simulink model "vipwarningsigns"  (R2017b)
settings: Solver=FixedStepDiscrete  StartTime=0  StopTime=inf  RelTol=1e-3  EnableMultiTasking=on
InitFcn:
  | % Maximum number of signs in a single frame
  | maxNumSigns=9;
  | % The .mat file reference below was generated using vipwarningsigns_templates.m
  | load vipwarningsigns_templates.mat;
model workspace (MATLAB code in the model file):
  | MaxBlkWidth=80;
undefined symbols (not defined in the file or in its folder): gray, Rec, SDTV, strel, template_detection, template_detection_display, template_ids, template_names, template_recognition, template_recognition_display
libraries: simulink x4, visiontextngfix x3, visionstatistics x1, visionmorphops x1, vipmisc x1, visionconversions x1, dspvision x1
CloseFcn:
  | clear maxNumSigns;
  | clear template_detection;
  | clear template_detection_display;
  | clear template_ids;
  | clear template_names;
  | clear template_recognition;
  | clear template_recognition_display;
settings Model: FPTRunName=Active  ExtModeAutoUpdateStatusClock=off  Creator=The MathWorks, Inc.  LastModifiedBy=The MathWorks, Inc.
settings DataIOCC: LimitDataPoints=on  SaveFormat=Array  SaveOutput=off  SignalLogging=off  SaveTime=off
settings OptimizationCC: ExpressionDepthLimit=2147483647  InitFltsAndDblsToZero=on  EfficientMapNaN2IntZero=off  LifeSpan=inf
settings DebuggingCC: UnderspecifiedInitializationDetection=Classic  MergeDetectMultiDrivingBlocksExec=none  SignalResolutionControl=TryResolveAllWithWarning  SolverPrmCheckMsg=warning  MultiTaskDSMMsg=warning  MultiTaskCondExecSysMsg=none  SigSpecEnsureSampleTimeMsg=none  ParameterPrecisionLossMsg=none  FcnCallInpInsideContextMsg=warning  AllowSymbolicDim=off  StateNameClashWarn=warning  SFUnexpectedBacktrackingDiag=warning  SFNoUnconditionalDefaultTransitionDiag=warning  SFExecutionAtInitializationDiag=none
settings HardwareCC: ProdBitPerPointer=32  ProdBitPerSizeT=32  ProdBitPerPtrDiffT=32  ProdLargestAtomicFloat=None  ProdIntDivRoundTo=Undefined  ProdEndianess=Unspecified  ProdWordSize=32  ProdHWDeviceType=32-bit Generic
settings ModelReferenceCC: PropagateSignalLabelsOutOfModel=off
settings SFSimCC: SimParseCustomCode=off
settings CodeAppCC: StateflowObjectComments=on
settings GRTTargetCC: TargetLangStandard=C89/C90 (ANSI)  GeneratePreprocessorConditionals=Disable all  CombineOutputUpdateFcns=off  GRTInterface=on
settings ConfigComp: CovMetricSettings=dw  CovHtmlReporting=on  CovSaveCumulativeToWorkspaceVar=on  CovSaveSingleToWorkspaceVar=on  CovExternalEMLEnable=off

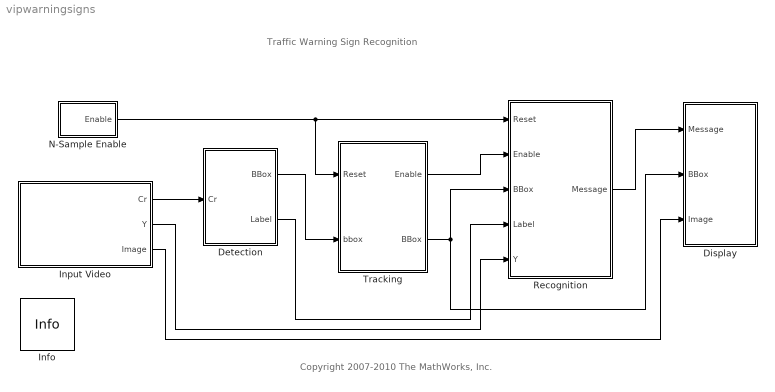
== system vipwarningsigns ==
  note: Traffic Warning Sign Recognition
  note: Copyright 2007-2010 The MathWorks, Inc.
  Detection : Subsystem
  Display : Subsystem
  Info : vipmisc/Info  SystemSampleTime=-1
      settings: SourceProductName=Computer Vision System Toolbox  SourceProductBaseCode=VP
  Input Video : Subsystem
      mask Display:
      | disp('vipwarnsigns.avi');
      | port_label('output',1,'Cr');
      | port_label('output',2,'Y');
      | port_label('output',3,'Image');
  N-Sample Enable : Subsystem  mask{sample=1}
      mask prompts: sample "Trigger Count, N"
  Recognition : Subsystem
  Tracking : Subsystem
  wires:
  Detection/1(BBox) -> Tracking/2(bbox)
  Input Video/1(Cr) -> Detection/1(Cr)
  N-Sample Enable/1(Enable) -> Tracking/1(Reset), Recognition/1(Reset)
  Tracking/1(Enable) -> Recognition/2(Enable)
  Tracking/2(BBox) -> Recognition/3(BBox), Display/2(BBox)
  Detection/2(Label) -> Recognition/4(Label)
  Input Video/2(Y) -> Recognition/5(Y)
  Recognition/1(Message) -> Display/1(Message)
  Input Video/3(Image) -> Display/3(Image)

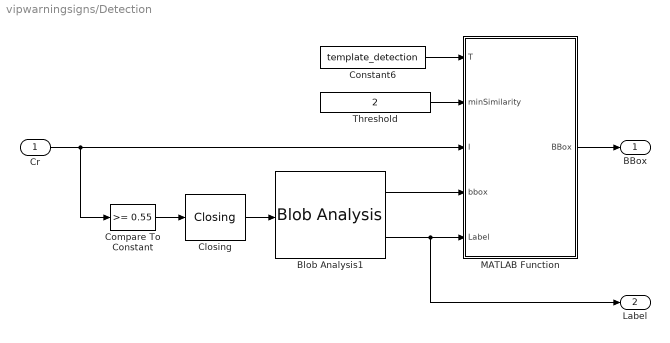
== system vipwarningsigns/Detection ==
  Cr : Inport
  Blob Analysis1 : visionstatistics/Blob Analysis  Tag=vipblks_row_conv  area=off  centroid=off  bBox=on  majorAxis=off  minorAxis=off  angle=off  eccentricity=off  equivDiameterSq=off  extent=off  perimeter=off  maxBlobs=maxNumSigns  warnIfNumBlobsExceeded=on  isCount=off  useMinArea=off  minArea=0  useMaxArea=off  maxArea=intmax('uint32')  excludeBorderBlob=off  outDT=double  isOutVarDim=on  isFill=on  fillValues=-1  conn=8  isLabel=on  outputMode=Binary point scaling  outputWordLength=32  outputFracLength=16  firstCoeffMode=Binary point scaling  firstCoeffWordLength=16  firstCoeffFracLength=14  secondCoeffMode=Binary point scaling  secondCoeffWordLength=32  secondCoeffFracLength=16  accumMode=Binary point scaling  accumWordLength=32  accumFracLength=0  prodOutputMode=Binary point scaling  prodOutputWordLength=32  prodOutputFracLength=16  roundingMode=Floor  overflowMode=off
      settings: SourceProductName=Computer Vision System Toolbox
  Closing : visionmorphops/Closing  nhoodsrc=Specify via dialog  strel=strel('rectangle', [15 15])
      settings: SourceProductName=Computer Vision System Toolbox  SourceProductBaseCode=VP
  Compare To Constant : simulink/Logic and Bit Operations/Compare To Constant  relop=>=  const=0.55  OutDataTypeStr=boolean  ZeroCross=off
  Constant6 : Constant  Value=template_detection  OutDataTypeStr=single
  MATLAB Function : MATLAB Function  TreatAsAtomicUnit=on
  Threshold : Constant  Value=2  OutDataTypeStr=single
  BBox : Outport
  Label : Outport  Port=2
  wires:
  Cr/1 -> MATLAB Function/3(I), Compare To Constant/1
  Closing/1 -> Blob Analysis1/1
  MATLAB Function/1(BBox) -> BBox/1
  Constant6/1 -> MATLAB Function/1(T)
  Blob Analysis1/2 -> MATLAB Function/5(Label), Label/1
  Compare To Constant/1 -> Closing/1
  Threshold/1 -> MATLAB Function/2(minSimilarity)
  Blob Analysis1/1 -> MATLAB Function/4(bbox)

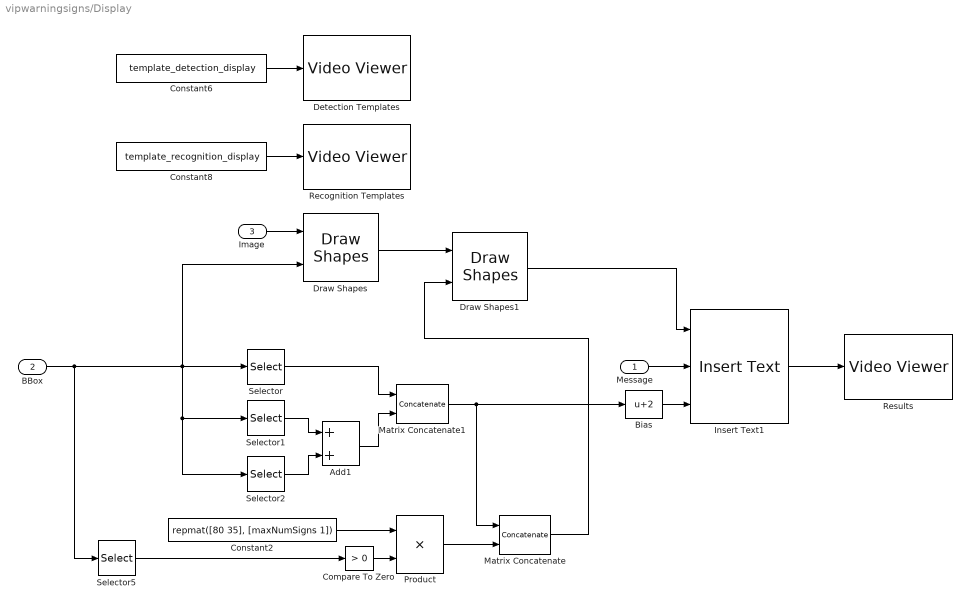
== system vipwarningsigns/Display ==
  Message : Inport
  BBox : Inport  Port=2
  Image : Inport  Port=3
  Add1 : Sum
  Bias : Bias  Bias=2
  Compare To Zero : simulink/Logic and Bit Operations/Compare To Zero  relop=>  OutDataTypeStr=uint8  ZeroCross=off
  Constant2 : Constant  Value=repmat([80 35], [maxNumSigns 1])  VectorParams1D=off  OutDataTypeStr=single
  Constant6 : Constant  Value=template_detection_display  OutDataTypeStr=single
  Constant8 : Constant  Value=template_recognition_display  OutDataTypeStr=single
  Detection Templates : VideoViewer  colormapValue=gray(256)  FigPos=[200 158 371 65]
  Draw Shapes : visiontextngfix/Draw Shapes  shape=Rectangles  fill=off  lineWidth=1  fillClrSource=Specify via dialog  display=User-specified value  intensity=200  color=[1 1 0]  opacity=0.6  viewport=Entire image  antialiasing=off  inType=Obsolete  imagePorts=One multidimensional signal  prodOutputMode=Binary point scaling  prodOutputWordLength=32  prodOutputFracLength=14  memoryMode=Specify word length  memoryWordLength=16  memoryFracLength=15  roundingMode=Floor  overflowMode=off
      settings: SourceProductName=Computer Vision System Toolbox
  Draw Shapes1 : visiontextngfix/Draw Shapes  shape=Rectangles  fill=on  lineWidth=1  fillClrSource=Specify via dialog  display=User-specified value  intensity=200  color=single([0 0 0])  opacity=single(1)  viewport=Entire image  antialiasing=off  inType=Obsolete  imagePorts=One multidimensional signal  prodOutputMode=Binary point scaling  prodOutputWordLength=32  prodOutputFracLength=14  memoryMode=Specify word length  memoryWordLength=16  memoryFracLength=14  roundingMode=Floor  overflowMode=off
      settings: SourceProductName=Computer Vision System Toolbox
  Insert Text1 : visiontextngfix/Insert Text  inputType=Obsolete  theText='%s'  getTextLocFrom=Input port  textLoc=[0 0]  getTextColorFrom=Specify via dialog  textColor=[1 0 0]'  getTextIntensityFrom=Specify via dialog  textIntensity=0  getTextOpacityFrom=Specify via dialog  textOpacity=1.0  dummyVar2=0  dummyVar3=0  dummyVar4=0  imagePorts=One multidimensional signal  isInputTransposed=off  fontFace=LucidaSansRegular  dummyVar1=0  blockFontSize=12  antiAliased=on
      settings: SourceProductName=Computer Vision System Toolbox  SourceProductBaseCode=VP
  Matrix Concatenate : Concatenate  Mode=Multidimensional array  ConcatenateDimension=2
  Matrix Concatenate1 : Concatenate  Mode=Multidimensional array  ConcatenateDimension=2
  Product : Product  RndMeth=Zero
  Recognition Templates : VideoViewer  colormapValue=gray(256)  FigPos=[200 325 371 88]
  Results : VideoViewer  colormapValue=gray(256)  FigPos=[585 365 410 238]
  Selector : Selector  NumberOfDimensions=2  InputPortWidth=4  IndexOptions=Select all,Index vector (dialog)  Indices=1,1  OutputSizes=1,1
  Selector1 : Selector  NumberOfDimensions=2  InputPortWidth=4  IndexOptions=Select all,Index vector (dialog)  Indices=3,2  OutputSizes=1,1
  Selector2 : Selector  NumberOfDimensions=2  InputPortWidth=4  IndexOptions=Select all,Index vector (dialog)  Indices=2,4  OutputSizes=1,1
  Selector5 : Selector  NumberOfDimensions=2  InputPortWidth=4  IndexOptions=Select all,Index vector (dialog)  Indices=[3 4],[3 4]  OutputSizes=1,1
  wires:
  Message/1 -> Insert Text1/2
  Image/1 -> Draw Shapes/1
  Insert Text1/1 -> Results/1
  Bias/1 -> Insert Text1/3
  Constant6/1 -> Detection Templates/1
  Constant8/1 -> Recognition Templates/1
  Selector/1 -> Matrix Concatenate1/1
  Selector1/1 -> Add1/1
  Draw Shapes/1 -> Draw Shapes1/1
  Draw Shapes1/1 -> Insert Text1/1
  Matrix Concatenate1/1 -> Bias/1, Matrix Concatenate/1
  Product/1 -> Matrix Concatenate/2
  Matrix Concatenate/1 -> Draw Shapes1/2
  Compare To Zero/1 -> Product/2
  Constant2/1 -> Product/1
  Selector5/1 -> Compare To Zero/1
  BBox/1 -> Selector5/1, Selector1/1, Selector2/1, Selector/1, Draw Shapes/2
  Selector2/1 -> Add1/2
  Add1/1 -> Matrix Concatenate1/2

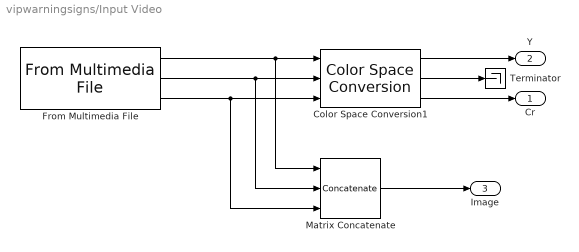
== system vipwarningsigns/Input Video ==
  Color Space Conversion1 : visionconversions/Color Space  Conversion  conversion=Obsolete  conversionActive=R'G'B' to Y'CbCr  wp_str=D65  rec=Rec. 601 (SDTV)  sys=1125/60/2:1  imagePorts=Separate color signals
      settings: SourceProductName=Computer Vision System Toolbox
  From Multimedia File : dspvision/From Multimedia File  inputFilename=vipwarnsigns.avi  loop=on  numPlays=inf  outputStreams=Video and audio  videoDataType=single  audioDataType=int16  inheritSampleTime=on  userDefinedSampleTime=1/30  noAudioOutput=off  isIntensityVideo=off  fourcc=RGB  colorVideoFormat=Separate color signals  outputEOF=off  dataOrg=Column-major  audioFrameSize=1024  computeAudioFrameSize=off  outSamplingMode=Frame based
      settings: SourceProductBaseCode=VP
  Matrix Concatenate : Concatenate  NumInputs=3  Mode=Multidimensional array  ConcatenateDimension=3
  Terminator : Terminator
  Cr : Outport
  Y : Outport  Port=2
  Image : Outport  Port=3
  wires:
  From Multimedia File/1 -> Color Space Conversion1/1, Matrix Concatenate/1
  From Multimedia File/2 -> Color Space Conversion1/2, Matrix Concatenate/2
  From Multimedia File/3 -> Color Space Conversion1/3, Matrix Concatenate/3
  Color Space Conversion1/1 -> Y/1
  Color Space Conversion1/2 -> Terminator/1
  Color Space Conversion1/3 -> Cr/1
  Matrix Concatenate/1 -> Image/1

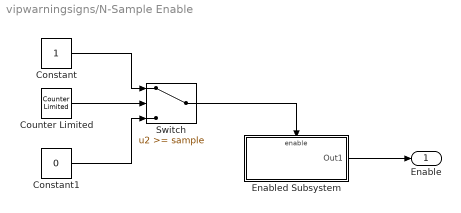
== system vipwarningsigns/N-Sample Enable ==
  Constant : Constant  OutDataTypeStr=boolean
  Constant1 : Constant  Value=0  OutDataTypeStr=boolean
  Counter Limited : simulink/Sources/Counter Limited  uplimit=sample  tsamp=-1
  Enabled Subsystem : Subsystem  TreatAsAtomicUnit=on
  Switch : Switch  Threshold=sample
  Enable : Outport
  wires:
  Counter Limited/1 -> Switch/2
  Constant1/1 -> Switch/3
  Constant/1 -> Switch/1
  Switch/1 -> Enabled Subsystem/Enable
  Enabled Subsystem/1(Out1) -> Enable/1

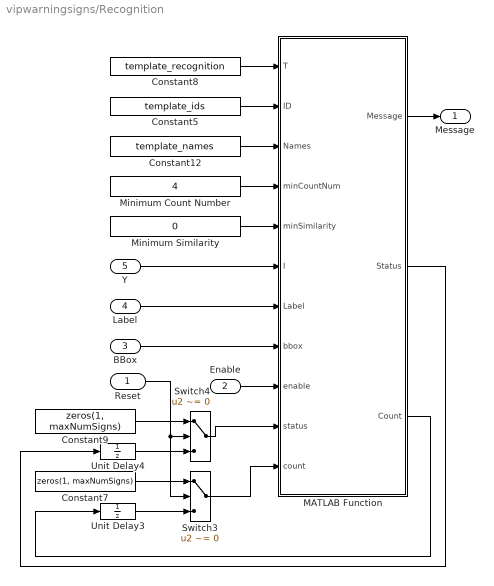
== system vipwarningsigns/Recognition ==
  Reset : Inport
  Enable : Inport  Port=2
  BBox : Inport  Port=3
  Label : Inport  Port=4
  Y : Inport  Port=5
  Constant12 : Constant  Value=template_names  OutDataTypeStr=single
  Constant5 : Constant  Value=template_ids  OutDataTypeStr=single
  Constant7 : Constant  Value=zeros(1, maxNumSigns)  OutDataTypeStr=single
  Constant8 : Constant  Value=template_recognition  OutDataTypeStr=single
  Constant9 : Constant  Value=zeros(1, maxNumSigns)  OutDataTypeStr=single
  MATLAB Function : MATLAB Function  TreatAsAtomicUnit=on
  Minimum Count Number : Constant  Value=4  OutDataTypeStr=single
  Minimum Similarity : Constant  Value=0  OutDataTypeStr=single
  Switch3 : Switch  Criteria=u2 ~= 0  OutDataTypeStr=Inherit: Inherit via back propagation  InputSameDT=on
  Switch4 : Switch  Criteria=u2 ~= 0  OutDataTypeStr=Inherit: Inherit via back propagation  InputSameDT=on
  Unit Delay3 : UnitDelay  SampleTime=-1
  Unit Delay4 : UnitDelay  SampleTime=-1
  Message : Outport
  wires:
  Constant8/1 -> MATLAB Function/1(T)
  Enable/1 -> MATLAB Function/9(enable)
  Y/1 -> MATLAB Function/6(I)
  MATLAB Function/1(Message) -> Message/1
  Reset/1 -> Switch3/2, Switch4/2
  BBox/1 -> MATLAB Function/8(bbox)
  Label/1 -> MATLAB Function/7(Label)
  Constant5/1 -> MATLAB Function/2(ID)
  Constant12/1 -> MATLAB Function/3(Names)
  MATLAB Function/2(Status) -> Unit Delay4/1
  Switch4/1 -> MATLAB Function/10(status)
  Unit Delay4/1 -> Switch4/3
  Constant9/1 -> Switch4/1
  MATLAB Function/3(Count) -> Unit Delay3/1
  Switch3/1 -> MATLAB Function/11(count)
  Unit Delay3/1 -> Switch3/3
  Constant7/1 -> Switch3/1
  Minimum Count Number/1 -> MATLAB Function/4(minCountNum)
  Minimum Similarity/1 -> MATLAB Function/5(minSimilarity)

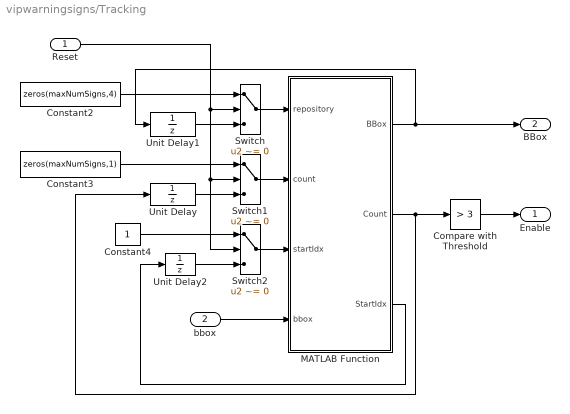
== system vipwarningsigns/Tracking ==
  Reset : Inport
  bbox : Inport  Port=2
  Compare with Threshold : simulink/Logic and Bit Operations/Compare To Constant  relop=>  const=3  OutDataTypeStr=boolean  ZeroCross=off
  Constant2 : Constant  Value=zeros(maxNumSigns,4)  OutDataTypeStr=single
  Constant3 : Constant  Value=zeros(maxNumSigns,1)  OutDataTypeStr=single
  Constant4 : Constant  OutDataTypeStr=single
  MATLAB Function : MATLAB Function  TreatAsAtomicUnit=on
  Switch : Switch  Criteria=u2 ~= 0  Threshold=1  OutDataTypeStr=Inherit: Inherit via back propagation  InputSameDT=on
  Switch1 : Switch  Criteria=u2 ~= 0  InputSameDT=on
  Switch2 : Switch  Criteria=u2 ~= 0  InputSameDT=on
  Unit Delay : UnitDelay  SampleTime=-1
  Unit Delay1 : UnitDelay  SampleTime=-1
  Unit Delay2 : UnitDelay  SampleTime=-1
  Enable : Outport
  BBox : Outport  Port=2
  wires:
  bbox/1 -> MATLAB Function/4(bbox)
  Compare with Threshold/1 -> Enable/1
  Reset/1 -> Switch2/2, Switch1/2, Switch/2
  Switch2/1 -> MATLAB Function/3(startIdx)
  MATLAB Function/3(StartIdx) -> Unit Delay2/1
  Unit Delay2/1 -> Switch2/3
  Constant4/1 -> Switch2/1
  Constant3/1 -> Switch1/1
  Unit Delay/1 -> Switch1/3
  MATLAB Function/2(Count) -> Compare with Threshold/1, Unit Delay/1
  MATLAB Function/1(BBox) -> BBox/1, Unit Delay1/1
  Unit Delay1/1 -> Switch/3
  Constant2/1 -> Switch/1
  Switch1/1 -> MATLAB Function/2(count)
  Switch/1 -> MATLAB Function/1(repository)

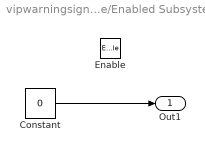
== system vipwarningsigns/N-Sample Enable/Enabled Subsystem ==
  Enable : EnablePort
  Constant : Constant  Value=0  OutDataTypeStr=boolean
  Out1 : Outport  InitialOutput=1
  wires:
  Constant/1 -> Out1/1

== matlab function vipwarningsigns/Tracking/MATLAB Function ==
  data: BBox output; repository input; count input; startIdx input; bbox input; Count output; StartIdx output; maxNumSigns parameter single size=1
function [BBox, Count, StartIdx] = Match(repository, count, startIdx, bbox, maxNumSigns)
% This function matches the targets found in the current video frame with
% those found in the previous frame. Targets in two video frames match
% when their bounding boxes overlap.
%
% Input:
%    repository: 
%       Bounding boxes of the targets found in the previous
%       frame. Each column has the format of [r, c, h, w] and corresponds 
%       to a target.
%    count: 
%       Number of video frames the target in the previous frame has 
%       been found.
%    startIdx: 
%       Index for the first new target in the current frame.
%    bbox: 
%       Bounding boxes of the targets found in the current frame.
%
% Output:
%    BBox: 
%       Bounding boxes of the targets found in the current frame. They
%       are ordered to have the same indices as their matching ones in the
%       previous frame.
%    Count: 
%       Number of video frames the target in the current frame has 
%       been found.
%    StartIdx: 
%       Index for the first new target in the next frame.

numBBox = single(size(bbox, 1));
BBox = single(zeros(maxNumSigns, 4));
Count = single(zeros(maxNumSigns,1));
impossible = single(10000); % A very large value
thr = single(2);
disMatrix = single(ones(maxNumSigns, numBBox)) * impossible;

% Calculate the distances between the repository and the current targets
for idx = single(1): maxNumSigns
    if repository(idx,3)>0 && repository(idx,4)>0
        for jdx = 1: numBBox
            if bbox(jdx,3)>0 && bbox(jdx,4)>0
                disMatrix(idx, jdx)...
                    = single(abs(2*(repository(idx,1)-bbox(jdx,1))...
                        +repository(idx,3)-bbox(jdx,3))...
                        / (repository(idx,3)+bbox(jdx,3))...
                        + abs(2*(repository(idx,2)-bbox(jdx,2))...
                        +repository(idx,4)-bbox(jdx,4))...
                        / (repository(idx,4)+bbox(jdx,4)));
            end
        end
    end
end

% Find the most similar pair of corners
for n = single(1): numBBox
    minVal = impossible;
    minIdx = single(0);
    minJdx = single(0);
    for idx = 1: single(maxNumSigns)
        for jdx = 1: numBBox
            if disMatrix(idx, jdx) < minVal
                minVal = disMatrix(idx, jdx);
                minIdx = idx;
                minJdx = jdx;
            end
        end
    end
    
    % Move the targets in the current frame so they have the same ordering
    % as their matching ones in the previous frame.
    if minVal < thr
        disMatrix(minIdx, :) = impossible;
        disMatrix(:, minJdx) = impossible;
        BBox(minIdx,:) = bbox(minJdx,:);
        Count(minIdx) = count(minIdx) + 1;
        bbox(minJdx,:) = single(zeros(4, 1));
    else
        break;
    end
end

% Copy the new targets
StartIdx = startIdx;
for jdx = single(1): numBBox
    if bbox(jdx,3)>0
        while BBox(StartIdx,3)
            if StartIdx<maxNumSigns
                StartIdx = StartIdx + single(1);
            else
                StartIdx = single(1);
            end
        end
        BBox(StartIdx, :) = bbox(jdx,:);
        Count(StartIdx) = single(1);
        if StartIdx<maxNumSigns
            StartIdx = StartIdx + single(1);
        else
            StartIdx = single(1);
        end
    end
end

== matlab function vipwarningsigns/Recognition/MATLAB Function ==
  data: Message output; Status output; T input; ID input; Names input; minCountNum input; minSimilarity input; I input; Label input; bbox input; enable input; status input; count input; Count output
function [Message, Status, Count] = Recognition(T, ID, Names, ...
    minCountNum, minSimilarity, I, Label, bbox, enable, status, count)
% This function finds the targets that are similar to any of the 
% templates. Similarity measure is calculated by correlation.
%
% Input:
%    T: 
%       Templates. Size is M-by-N-by-K, where M and N are the number of
%       rows and the number of columns in each template, respectively.
%       K is the number of templates.
%    ID:
%       Target types of the templates. That is, a target may have several
%       templates, and ID indicates which templates correspond to the same
%       targets.
%    Names:
%       Names of the targets.
%    minCountNum: 
%       Minimum number of consecutive times the target must be recongized 
%       for it to be considered valid.
%    minSimilarity: 
%       Target similarity threshold.
%    I: 
%       Intensity image under test.
%    Label: 
%        Labeled image. Pixels from the same potential target have
%        the same label.
%    bbox: Bounding boxes of the potential targets. Each column has the
%        format of [r, c, h, w] and corresponds to a pontential target.
%    enable: 
%        Indicator of the valid potential targets.
%    status: 
%        Previous recognition results.
%    count: 
%        Previous correct recognition number.
%
% Output:
%    Message: 
%        Message for display.
%    Status: 
%        Recognition results indicating template matches.
%    Count: 
%        Vector containing number of times a particular target was
%        recognized.
%    BBox: 
%        Boudning boxes of the valid targets. 

numImgRows = single(size(Label, 1));
numImgCols = single(size(Label, 2));
numTmpRows = single(size(T, 1));
numTmpCols = single(size(T, 2));
numTemplates = single(size(T, 3));
numBBox = single(size(bbox, 1));
numChars = size(Names, 2);
lenNames = single(zeros(1, size(Names, 1)));
feature = single(zeros(numTmpRows, numTmpCols));
Message = uint8(zeros(1, numBBox*(numChars+6)));
Status = single(zeros(1, numBBox));
Count = single(zeros(1, numBBox));

% Calculate the length of target names
for idx = single(1): size(Names, 1)
    for jdx = numChars: -1: single(1)
        if Names(idx, jdx)
            lenNames(idx) = jdx;
            break;
        end
    end
end

for idx = single(1): numBBox
    bestID = single(0);
    bestConfidence = single(0);
    
    if enable(idx)==1
        if count(idx) > minCountNum
            Status(idx) = status(idx);
            Count(idx) = count(idx) + 1;

        else
            stepRows = floor(single(bbox(idx,4)) / numTmpRows);
            stepCols = floor(single(bbox(idx,3)) / numTmpCols);

            startColList = single(zeros(1, 3));
            startColList(2) = bbox(idx,1);
            startColList(1) = max(1, startColList(2)-stepCols);
            startColList(3) = min(numImgCols, startColList(2)+stepCols);

            endColList = single(zeros(1, 3));
            endColList(2) = bbox(idx,1)+bbox(idx,3)-1;
            endColList(1) = max(1, endColList(2)-stepCols);
            endColList(3) = min(numImgCols, endColList(2)+stepCols);

            startRowList = single(zeros(1, 3));
            startRowList(2) = bbox(idx,2);
            startRowList(1) = max(1, startRowList(2)-stepRows);
            startRowList(3) = min(numImgRows, startRowList(2)+stepRows);

            endRowList = single(zeros(1, 3));
            endRowList(2) = bbox(idx,2)+bbox(idx,4)-1;
            endRowList(1) = max(1, endRowList(2)-stepRows);
            endRowList(3) = min(numImgRows, endRowList(2)+stepRows);

            for startCol = startColList
                for endCol = endColList
                    ratioCols = (endCol - startCol) / numTmpCols;
                    for startRow = startRowList
                        for endRow = endRowList
                            ratioRows = (endRow - startRow) / numTmpRows;

                            % Calculate features
                            colSrcFlt = startCol;
                            for col = 1: numTmpCols
                                colSrc = floor(colSrcFlt);
                                rowSrcFlt = startRow;
                                for row = 1: numTmpRows
                                    rowSrc = floor(rowSrcFlt);
                                    feature(row, col) = I(rowSrc,colSrc);
                                    rowSrcFlt = rowSrcFlt + ratioRows;
                                end
                                colSrcFlt = colSrcFlt + ratioCols;
                            end

                            % Normalization
                            feature = feature - mean(feature(:));

                            % Matching
                            for iTmp = 1: numTemplates
                                confidence = single(0);
                                for col = 1: numTmpCols
                                    for row = 1: numTmpRows
                                        confidence = confidence ...
                                            + T(row,col,iTmp)*feature(row,col);
                                    end
                                end
                                if confidence > bestConfidence
                                    bestConfidence = confidence;
                                    bestID = ID(iTmp);
                                end
                            end
                        end
                    end
                end
            end

            if bestConfidence>=minSimilarity
                if status(idx)==bestID;
                    Count(idx) = count(idx) + 1;
                else
                    Count(idx) = 1;
                end
                Status(idx) = bestID;
            end
        end
    end
end

% Generate output messages
iMessage = single(1);
for idx = single(1): numBBox
    if Count(idx)>=minCountNum || enable(idx)==1
        bestID = Status(idx);
        if Count(idx)>=minCountNum
            % Display target name
            for jdx = single(1): lenNames(bestID)
                Message(iMessage+jdx-1) = Names(bestID, jdx);
            end
            iMessage = iMessage + lenNames(bestID);
        else
            Message(iMessage)   = uint8('R');
            Message(iMessage+1) = uint8('e');
            Message(iMessage+2) = uint8('c');
            Message(iMessage+3) = uint8('o');
            Message(iMessage+4) = uint8('g');
            Message(iMessage+5) = uint8('n');
            Message(iMessage+6) = uint8('i');
            Message(iMessage+7) = uint8('z');
            Message(iMessage+8) = uint8('e');
            Message(iMessage+9) = uint8('.');
            Message(iMessage+10) = uint8('.');
            Message(iMessage+11) = uint8('.');
            iMessage = iMessage + single(12);
        end
        
        % Display Tag
        Message(iMessage)   = uint8(10);  % '\n'
        Message(iMessage+1) = uint8('T');
        Message(iMessage+2) = uint8('a');
        Message(iMessage+3) = uint8('g');
        Message(iMessage+4) = uint8(':');
        Message(iMessage+5) = uint8('0'+idx);
        iMessage = iMessage + single(6);
    end
    iMessage = iMessage + single(1);
end

== matlab function vipwarningsigns/Detection/MATLAB Function ==
  data: BBox output size=[9 4]; T input; minSimilarity input; I input; bbox input; Label input
function BBox = Detection(T, minSimilarity, I, bbox, Label)
% This function finds the targets that are similar enough to any of the 
% templates. Similarity measure is calculated by correlation.
%
% Input:
%    T: 
%       Templates. Size is M-by-N-by-K, where M and N are the number of
%       rows and the number of columns in each template, respectively.
%       K is the number of templates.
%    minSimilarity: 
%       The minimum similarity a potential target and any of 
%       the templates must have in order for the blob to be considered as 
%       a valid target.
%    I: 
%       Intensity image under test.
%    bbox: 
%       Bounding boxes of the potential targets. Each column has the
%       format of [r, c, h, w] and corresponds to a pontential target.
%    Label: 
%       Labeled image. Pixels from the same potential target have
%       the same label.
%
% Output:
%    BBox: 
%       Bounding boxes of the valid targets. 

numImgRows = single(size(Label, 2));
numImgCols = single(size(Label, 1));
numTmpRows = single(size(T, 1));
numTmpCols = single(size(T, 2));
numTemplates = single(size(T, 3));
numBBox = single(size(bbox, 1));
feature = single(zeros(numTmpRows, numTmpCols));
BBox = single(zeros(numBBox,4));


for idx = 1: numBBox
    bestSimilarity = single(0);
    
    if bbox(idx,4)>=numTmpRows && bbox(idx,3)>=numTmpCols
        % Step sizes for calculating features
        stepRows = floor(single(bbox(idx,4)) / numTmpRows);
        stepCols = floor(single(bbox(idx,3)) / numTmpCols);
        
        % Each side of the bounding box has been tried on three different
        % positions.
        startColList = single(zeros(1, 3));
        startColList(2) = bbox(idx,1);
        startColList(1) = max(1, startColList(2)-stepCols);
        startColList(3) = min(numImgCols, startColList(2)+stepCols);
        
        endColList = single(zeros(1, 3));
        endColList(2) = bbox(idx,1)+bbox(idx,3)-1;
        endColList(1) = max(1, endColList(2)-stepCols);
        endColList(3) = min(numImgCols, endColList(2)+stepCols);
        
        startRowList = single(zeros(1, 3));
        startRowList(2) = bbox(idx,2);
        startRowList(1) = max(1, startRowList(2)-stepRows);
        startRowList(3) = min(numImgRows, startRowList(2)+stepRows);
        
        endRowList = single(zeros(1, 3));
        endRowList(2) = bbox(idx,2)+bbox(idx,4)-1;
        endRowList(1) = max(1, endRowList(2)-stepRows);
        endRowList(3) = min(numImgRows, endRowList(2)+stepRows);
        
        % Try all possible positions for bouding box and find the best match
        for startCol = startColList
            for endCol = endColList
                ratioCols = (endCol - startCol) / numTmpCols;
                for startRow = startRowList
                    for endRow = endRowList
                        ratioRows = (endRow - startRow) / numTmpRows;
                        
                        % Calculate features
                        colSrcFlt = startCol;
                        for col = 1: numTmpCols
                            colSrc = floor(colSrcFlt);
                            rowSrcFlt = startRow;
                            for row = 1: numTmpRows
                                rowSrc = floor(rowSrcFlt);
                                feature(row, col) = I(rowSrc,colSrc);
                                rowSrcFlt = rowSrcFlt + ratioRows;
                            end
                            colSrcFlt = colSrcFlt + ratioCols;
                        end
                        
                        % Normalization
                        feature = feature - mean(feature(:));
                            
                        % Match with each of the templates
                        for iTmp = 1: numTemplates
                            similarity = single(0);
                            % Correlation
                            for col = 1: numTmpCols
                                for row = 1: numTmpRows
                                    similarity = similarity ...
                                        + T(row,col,iTmp)*feature(row,col);
                                end
                            end
                            if similarity > bestSimilarity
                                bestSimilarity = similarity;
                            end
                        end
                    end
                end
            end
        end
        
        % Output the valid targets
        if bestSimilarity>=minSimilarity
            BBox(idx,1) = bbox(idx,1);
            BBox(idx,2) = bbox(idx,2);
            BBox(idx,3) = bbox(idx,3);
            BBox(idx,4) = bbox(idx,4);
        end
    end
end
